simulink model "main"  (R2026a)
settings: Solver=ode45  StopTime=100  MaxStep=0.01
values from neighbouring files (symbols this model uses):
  A = 2.2    [constants.m]
  alpha_3 = alpha(3)    [constants.m]
  beta = 0.35    [constants.m]
  C_d = 0.36    [constants.m]
  C_r = 0.01    [constants.m]
  cancel = 0    [constants.m]
  g = 9.81    [constants.m]
  ideal_v_r = 30    [constants.m]
  k_i = 0.0075    [constants.m]
  k_p = 0.09    [constants.m]
  m = 1200    [constants.m]
  on_off = 0    [constants.m]
  resume_accel = 0    [constants.m]
  rho = 1.3    [constants.m]
  set_decel = 0    [constants.m]
  T_m = 200    [constants.m]
  theta = 0    [constants.m]
  w_m = 450    [constants.m]
settings Model: Creator=DELL  LastModifiedBy=DELL

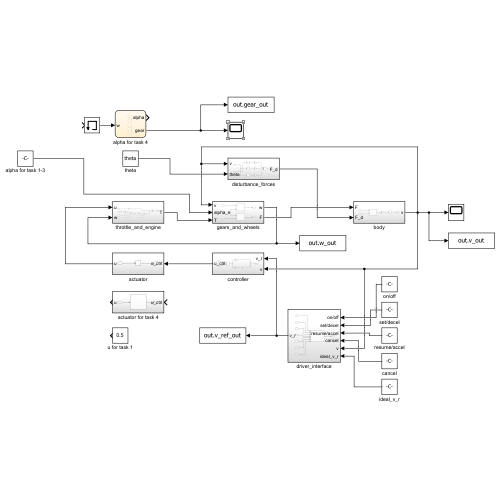
[thumbnail: Simulink's stored preview of the top-level diagram]
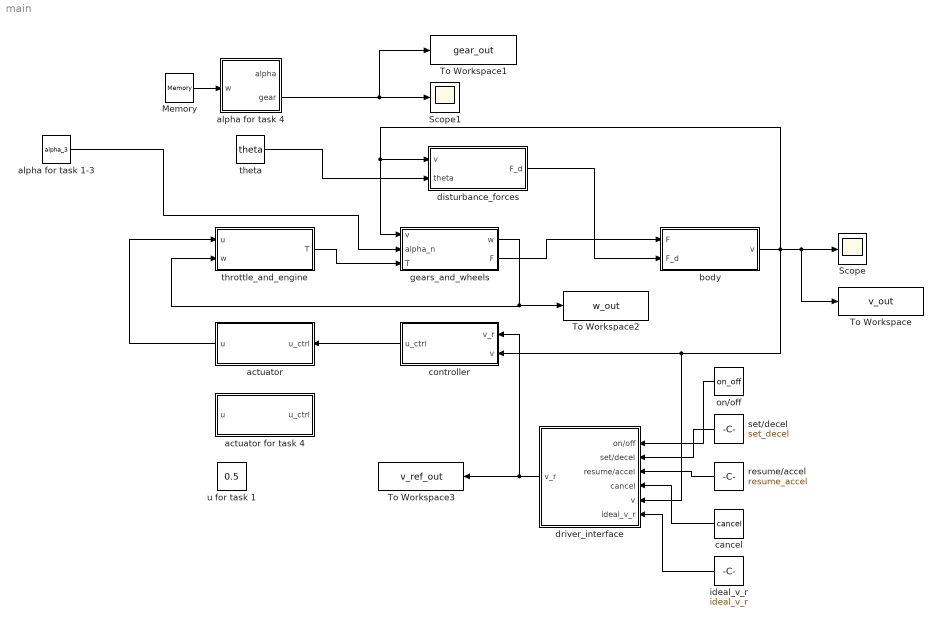
== system main ==
  Memory : Memory
  Scope : Scope
      settings: ActiveDisplayYMinimum=18.630360275102785  ActiveDisplayYMaximum=32.3142752983266
  Scope1 : Scope
      settings: ActiveDisplayYMinimum=0.87962205407173455  ActiveDisplayYMaximum=6.0075741233409117
  To Workspace : ToWorkspace  VariableName=v_out  SaveFormat=Structure With Time  SampleTime=-1
  To Workspace1 : ToWorkspace  VariableName=gear_out  SaveFormat=Structure With Time  SampleTime=-1
  To Workspace2 : ToWorkspace  VariableName=w_out  SaveFormat=Structure With Time  SampleTime=-1
  To Workspace3 : ToWorkspace  VariableName=v_ref_out  SaveFormat=Structure With Time  SampleTime=-1
  actuator : Subsystem
      settings: PortSchema="{\"entries\":[{\"content\":{\"sides\":[{\"content\":{\"connectorIds\":[\"Out1\"]},\"type\":\"ConnectorPlacement.EquallySpacedRectSide\",\"uuid\":\"1ed1fd3f-d9e8-489c-9ef6-29115445d832\"},{\"content\":{\"connectorIds\":[\"In1\"],\"side\":\"RIGHT\"},\"type\":\"ConnectorPlacement.EquallySpacedRectSide\",\"uuid\":\"cba28840-f4dd-4c82-8df2-502c6afdbda0\"},{\"content\":{\"side\":\"TOP\"},\"type\":\"ConnectorPlacement.EquallySpacedRectSide\",\"uuid\":\"27aaa382-ecb9-44b1-925e-36cfda6631f1\"}]},\"type\":\"ConnectorPlacement.EquallySpacedConnector\",\"uuid\":\"e8920326-9f6a-4dab-bf44-db418cdf5e32\"}],\"packageUris\":[\"http://schema.mathworks.com/mf0/Connector/R2020b\"],\"version\":\"1.0\"}"
  actuator for task 4 : Subsystem
  alpha for task 1-3 : Constant  Value=alpha_3
  alpha for task 4 : Stateflow chart  TreatAsAtomicUnit=on
  body : Subsystem
  cancel : Constant  Value=cancel
  controller : Subsystem
      settings: PortSchema="{\"entries\":[{\"content\":{\"sides\":[{\"content\":{\"connectorIds\":[\"Out1\"]},\"type\":\"ConnectorPlacement.EquallySpacedRectSide\",\"uuid\":\"553eb755-11bb-43c1-b4e4-68de2c64b51a\"},{\"content\":{\"connectorIds\":[\"In1\",\"In2\"],\"side\":\"RIGHT\"},\"type\":\"ConnectorPlacement.EquallySpacedRectSide\",\"uuid\":\"424a16fc-98c8-404c-b7fb-386b9e06adf4\"},{\"content\":{\"side\":\"TOP\"},\"type\":\"ConnectorPlacement.EquallySpacedRectSide\",\"uuid\":\"05f53437-ec27-48db-9993-03b089c6a791\"}]},\"type\":\"ConnectorPlacement.EquallySpacedConnector\",\"uuid\":\"3405b2ca-b482-436b-907d-54026e53ffb2\"}],\"packageUris\":[\"http://schema.mathworks.com/mf0/Connector/R2020b\"],\"version\":\"1.0\"}"
  disturbance_forces : Subsystem
  driver_interface : Subsystem
      settings: PortSchema="{\"entries\":[{\"content\":{\"sides\":[{\"content\":{\"connectorIds\":[\"Out1\"]},\"type\":\"ConnectorPlacement.EquallySpacedRectSide\",\"uuid\":\"1b3ba72c-0b75-4471-8fc8-ec093cc62009\"},{\"content\":{\"connectorIds\":[\"In1\",\"In2\",\"In3\",\"In4\",\"In5\",\"In6\"],\"side\":\"RIGHT\"},\"type\":\"ConnectorPlacement.EquallySpacedRectSide\",\"uuid\":\"9888d5fa-b32b-4147-b598-475b34976128\"},{\"content\":{\"side\":\"TOP\"},\"type\":\"ConnectorPlacement.EquallySpacedRectSide\",\"uuid\":\"54021165-6d42-436b-9749-1184e77cd3c2\"}]},\"type\":\"ConnectorPlacement.EquallySpacedConnector\",\"uuid\":\"275db26c-470c-4fc8-8b70-801213306570\"}],\"packageUris\":[\"http://schema.mathworks.com/mf0/Connector/R2020b\"],\"version\":\"1.0\"}"
  gears_and_wheels : Subsystem
  ideal_v_r : Constant  Value=ideal_v_r
  on/off : Constant  Value=on_off
  resume/accel : Constant  Value=resume_accel
  set/decel : Constant  Value=set_decel
  theta : Constant  Value=theta
  throttle_and_engine : Subsystem
  u for task 1 : Constant  Value=0.5
  wires:
  gears_and_wheels/2(F) -> body/1(F)
  disturbance_forces/1(F_d) -> body/2(F_d)
  throttle_and_engine/1(T) -> gears_and_wheels/3(T)
  body/1(v) -> To Workspace/1, Scope/1, driver_interface/5(v), controller/2(v), gears_and_wheels/1(v), disturbance_forces/1(v)
  theta/1 -> disturbance_forces/2(theta)
  gears_and_wheels/1(w) -> To Workspace2/1, throttle_and_engine/2(w)
  driver_interface/1(v_r) -> To Workspace3/1, controller/1(v_r)
  on/off/1 -> driver_interface/1(on/off)
  set/decel/1 -> driver_interface/2(set/decel)
  resume/accel/1 -> driver_interface/3(resume/accel)
  cancel/1 -> driver_interface/4(cancel)
  ideal_v_r/1 -> driver_interface/6(ideal_v_r)
  Memory/1 -> alpha for task 4/1(w)
  alpha for task 4/2(gear) -> To Workspace1/1, Scope1/1
  alpha for task 1-3/1 -> gears_and_wheels/2(alpha_n)
  actuator/1(u) -> throttle_and_engine/1(u)
  controller/1(u_ctrl) -> actuator/1(u_ctrl)

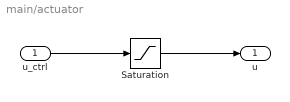
== system main/actuator ==
  u_ctrl : Inport
  Saturation : Saturate  UpperLimit=1  LowerLimit=0
  u : Outport
  wires:
  u_ctrl/1 -> Saturation/1
  Saturation/1 -> u/1

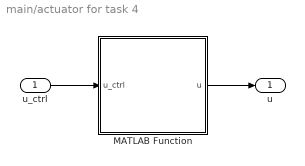
== system main/actuator for task 4 ==
  u_ctrl : Inport
  MATLAB Function : MATLAB Function  TreatAsAtomicUnit=on
  u : Outport
  wires:
  u_ctrl/1 -> MATLAB Function/1(u_ctrl)
  MATLAB Function/1(u) -> u/1

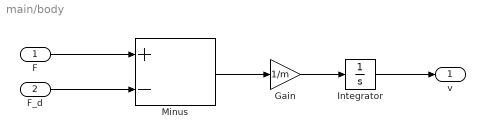
== system main/body ==
  F : Inport
  F_d : Inport  Port=2
  Gain : Gain  Gain=1/m
  Integrator : Integrator  InitialCondition=20
  Minus : Sum  Inputs=+-
  v : Outport
  wires:
  Minus/1 -> Gain/1
  F_d/1 -> Minus/2
  F/1 -> Minus/1
  Integrator/1 -> v/1
  Gain/1 -> Integrator/1

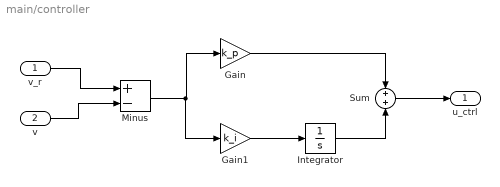
== system main/controller ==
  v_r : Inport
  v : Inport  Port=2
  Gain : Gain  Gain=k_p
  Gain1 : Gain  Gain=k_i
  Integrator : Integrator  InitialCondition=0.104
  Minus : Sum  Inputs=+-
  Sum : Sum
  u_ctrl : Outport
  wires:
  v_r/1 -> Minus/1
  v/1 -> Minus/2
  Minus/1 -> Gain1/1, Gain/1
  Gain/1 -> Sum/1
  Gain1/1 -> Integrator/1
  Sum/1 -> u_ctrl/1
  Integrator/1 -> Sum/2

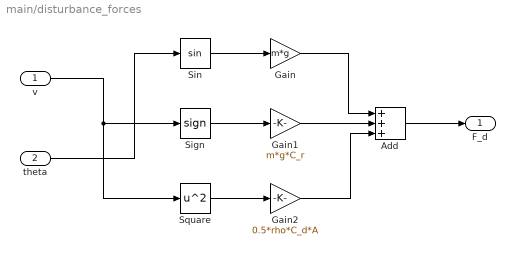
== system main/disturbance_forces ==
  v : Inport
  theta : Inport  Port=2
  Add : Sum  Inputs=+++
  Gain : Gain  Gain=m*g
  Gain1 : Gain  Gain=m*g*C_r
  Gain2 : Gain  Gain=0.5*rho*C_d*A
  Sign : Signum  ZeroCross=off
  Sin : Trigonometry
  Square : Math  Operator=square
  F_d : Outport
  wires:
  Add/1 -> F_d/1
  theta/1 -> Sin/1
  Sin/1 -> Gain/1
  Gain/1 -> Add/1
  v/1 -> Square/1, Sign/1
  Sign/1 -> Gain1/1
  Gain1/1 -> Add/2
  Square/1 -> Gain2/1
  Gain2/1 -> Add/3

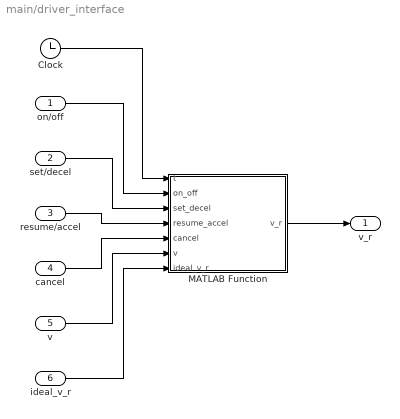
== system main/driver_interface ==
  on/off : Inport
  set/decel : Inport  Port=2
  resume/accel : Inport  Port=3
  cancel : Inport  Port=4
  v : Inport  Port=5
  ideal_v_r : Inport  Port=6
  Clock : Clock
  MATLAB Function : MATLAB Function  TreatAsAtomicUnit=on
  v_r : Outport
  wires:
  MATLAB Function/1(v_r) -> v_r/1
  on/off/1 -> MATLAB Function/2(on_off)
  set/decel/1 -> MATLAB Function/3(set_decel)
  resume/accel/1 -> MATLAB Function/4(resume_accel)
  cancel/1 -> MATLAB Function/5(cancel)
  v/1 -> MATLAB Function/6(v)
  ideal_v_r/1 -> MATLAB Function/7(ideal_v_r)
  Clock/1 -> MATLAB Function/1(t)

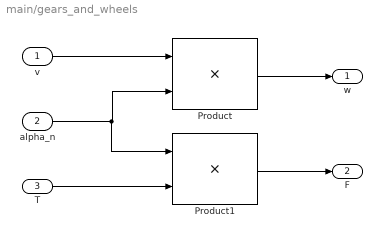
== system main/gears_and_wheels ==
  v : Inport
  alpha_n : Inport  Port=2
  T : Inport  Port=3
  Product : Product
  Product1 : Product
  w : Outport
  F : Outport  Port=2
  wires:
  T/1 -> Product1/2
  Product1/1 -> F/1
  Product/1 -> w/1
  alpha_n/1 -> Product1/1, Product/2
  v/1 -> Product/1

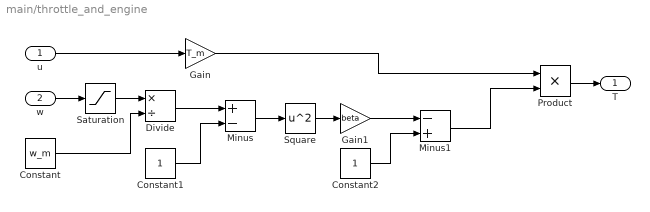
== system main/throttle_and_engine ==
  u : Inport
  w : Inport  Port=2
  Constant : Constant  Value=w_m
  Constant1 : Constant
  Constant2 : Constant
  Divide : Product  Inputs=*/
  Gain : Gain  Gain=T_m
  Gain1 : Gain  Gain=beta
  Minus : Sum  Inputs=+-
  Minus1 : Sum  Inputs=-+
  Product : Product
  Saturation : Saturate  UpperLimit=inf  LowerLimit=0.01
  Square : Math  Operator=square
  T : Outport  Unit=N*m
  wires:
  u/1 -> Gain/1
  Constant/1 -> Divide/2
  Square/1 -> Gain1/1
  Product/1 -> T/1
  w/1 -> Saturation/1
  Saturation/1 -> Divide/1
  Minus/1 -> Square/1
  Divide/1 -> Minus/1
  Constant1/1 -> Minus/2
  Constant2/1 -> Minus1/2
  Gain1/1 -> Minus1/1
  Minus1/1 -> Product/2
  Gain/1 -> Product/1

== matlab function main/actuator for task 4/MATLAB Function ==
  data: u_ctrl input; u output
function u = u_control(u_ctrl)
    u = 1;
end

== matlab function main/driver_interface/MATLAB Function ==
  data: t input; on_off input; v_r output; set_decel input; resume_accel input; cancel input; v input; ideal_v_r input
function v_r = driver(t, on_off, set_decel, resume_accel, cancel, v, ideal_v_r)
    if t < 10
        v_r = 20;
    else
        v_r = 30;
end

== stateflow chart main/alpha for task 4 ==
  state Gear1
    entry:
    alpha = 40;
    gear = 1;
  state Gear2
    entry:
    alpha = 25;
    gear = 2;
  state Gear3
    entry:
    alpha = 16;
    gear = 3;
  state Gear4
    entry:
    alpha = 12;
    gear = 4;
  state Gear5
    entry:
    alpha = 10;
    gear = 5;
  (default) -> Gear1
  Gear2 -> Gear1 [order 2] : [w<=220]
  Gear1 -> Gear2 : [w>=420]
  Gear3 -> Gear2 [order 2] : [w<=220]
  Gear2 -> Gear3 [order 1] : [w>=420]
  Gear4 -> Gear3 [order 2] : [w<=220]
  Gear3 -> Gear4 [order 1] : [w>=420]
  Gear5 -> Gear4 : [w<=220]
  Gear4 -> Gear5 [order 1] : [w>=420]
  data: w input; alpha output; gear output
